simulink model "dc_motor_control_PCI_16E4_2015a"  (R2020b)
settings: Solver=ode3  StartTime=0.0  StopTime=10  RelTol=1e-3
model workspace (MAT data in the model file):
  freq = 0
  tau = 1.51
values from neighbouring files (symbols this model uses):
  a = 37.04    [ControlSystemDesigner_e_Nyquist.m]    (also in ex3_5.m)
  k0 = 1.382    [ControlSystemDesigner_e_Nyquist.m]
  k1 = 6.9094    [ControlSystemDesigner_e_Nyquist.m]
  z = 14.89    [ControlSystemDesigner_e_Nyquist.m]    (also in ex3_5.m = 5)
undefined symbols (not defined in the file or in its folder): National_Instruments, PCI
libraries: sldrtlib x5
settings Model: SimulationMode=external  ExtModeTrigDuration=60001  Creator=Alunos  LastModifiedBy=rodsc
settings DataIOCC: LimitDataPoints=on  SaveFormat=Array  ReturnWorkspaceOutputs=off
settings OptimizationCC: BlockReduction=off  BooleanDataType=off
settings DebuggingCC: SaveWithParameterizedLinksMsg=none  UnderspecifiedInitializationDetection=Classic  MergeDetectMultiDrivingBlocksExec=none  SignalResolutionControl=TryResolveAllWithWarning  SFUnexpectedBacktrackingDiag=warning  SFNoUnconditionalDefaultTransitionDiag=warning  SFExecutionAtInitializationDiag=none  ArithmeticOperatorsInVariantConditions=warning
settings HardwareCC: TargetIntDivRoundTo=Zero  TargetEndianess=LittleEndian  TargetHWDeviceType=Intel->x86/Pentium
settings ModelReferenceCC: PropagateSignalLabelsOutOfModel=off
settings SFSimCC: SimUseLocalCustomCode=off  CustomCodeUndefinedFunction=UseInterfaceOnly
settings RTWCC: Description=Simulink Desktop Real-Time  SystemTargetFile=sldrt.tlc  TemplateMakefile=sldrt.tmf  RTWUseLocalCustomCode=off  RTWCompilerOptimization=on
settings CodeAppCC: MaxIdLength=95  StateflowObjectComments=on
settings SimulinkDesktopRealTimeCC: TargetPreCompLibLocation=C:\Program Files\Matlab\toolbox\sldrt\lib\win64  TargetLangStandard=C89/C90 (ANSI)  SupportVariableSizeSignals=off
settings ConfigComp: CovMetricSettings=dw  CovSaveCumulativeToWorkspaceVar=on  CovSaveSingleToWorkspaceVar=on  CovExternalEMLEnable=off

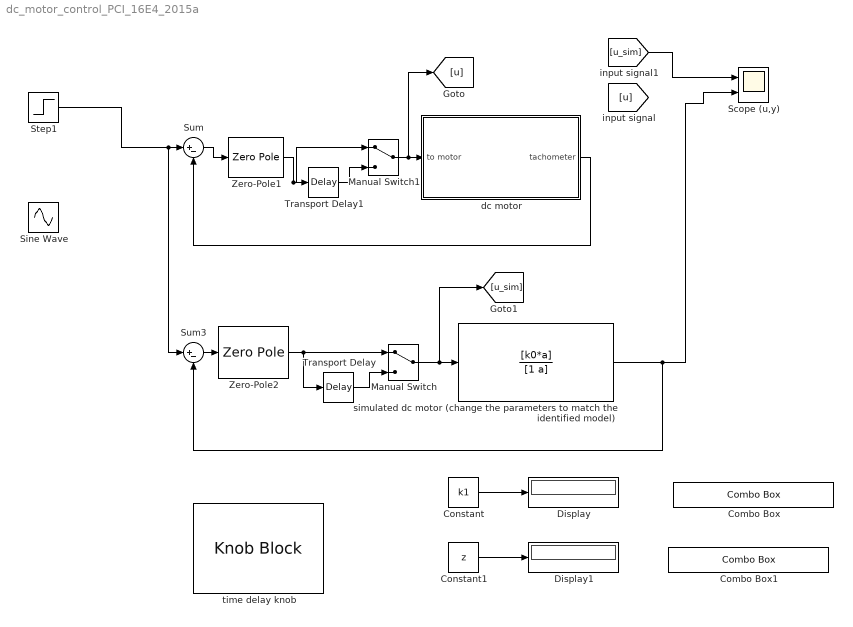
== system dc_motor_control_PCI_16E4_2015a ==
  Combo Box : ComboBox  LabelPosition=Hide  SelectedLabel=Label3
      settings: Values={{'Label1', 'Label2', 'Label3', 'default'}, [4 30 800 6.9094]}
  Combo Box1 : ComboBox  LabelPosition=Hide  SelectedLabel=Label2
      settings: Values={{'Label1', 'Label2', 'Label3', 'default'}, [4 50 150 14.89]}
  Constant : Constant  Value=k1
  Constant1 : Constant  Value=z
  Display : Display
  Display1 : Display
  Manual Switch : ManualSwitch
  Manual Switch1 : ManualSwitch
  Scope (u,y) : Scope  NumInputPorts=2
  Sine Wave : Sin  SampleTime=0
  Step1 : Step  Time=0.2  SampleTime=0
  Sum : Sum  Inputs=|+-
  Sum3 : Sum  Inputs=|+-
  Transport Delay : TransportDelay  DelayTime=tau  FixedBuffer=on  TransDelayFeedthrough=on
  Transport Delay1 : TransportDelay  DelayTime=tau  FixedBuffer=on  TransDelayFeedthrough=on
  Zero-Pole1 : ZeroPole  Zeros=[-z]  Poles=[0]  Gain=[k1/z]
  Zero-Pole2 : ZeroPole  Zeros=[-z]  Poles=0  Gain=[k1/z]
  dc motor : Subsystem
  simulated dc motor (change the parameters to match the identified model) : TransferFcn  Numerator=[k0*a]  Denominator=[1 a]
  time delay knob : KnobBlock  ScaleMax=0.150  TickInterval=0.1
  wires:
  simulated dc motor (change the parameters to match the identified model)/1 -> Scope (u,y)/2, Sum3/2
  Sum/1 -> Zero-Pole1/1
  Zero-Pole2/1 -> Transport Delay/1, Manual Switch/1
  [u_sim] -> Scope (u,y)/1
  Sum3/1 -> Zero-Pole2/1
  dc motor/1(tachometer) -> Sum/2
  Manual Switch/1 -> [u_sim], simulated dc motor (change the parameters to match the identified model)/1
  Transport Delay/1 -> Manual Switch/2
  Zero-Pole1/1 -> Manual Switch1/1, Transport Delay1/1
  Transport Delay1/1 -> Manual Switch1/2
  Manual Switch1/1 -> [u], dc motor/1(to motor)
  Step1/1 -> Sum3/1, Sum/1
  Constant1/1 -> Display1/1
  Constant/1 -> Display/1

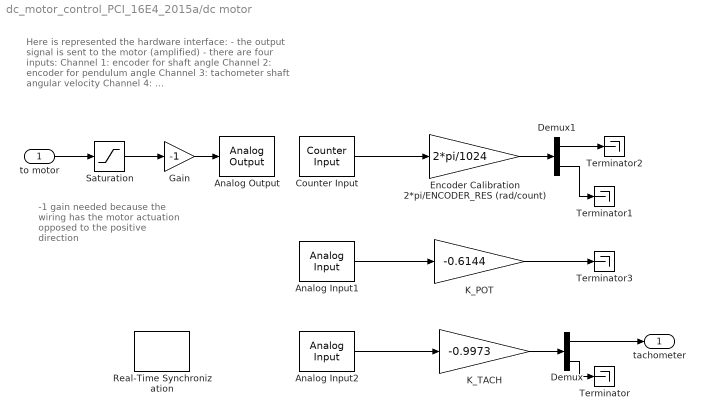
== system dc_motor_control_PCI_16E4_2015a/dc motor ==
  note: -1 gain needed
      | because the wiring
      | has the motor
      | actuation opposed to
      | the positive direction
  note: Here is represented the hardware interface:
      | - the output signal is sent to the motor (amplified)
      | - there are four inputs:
      | Channel 1: encoder for shaft angle
      | Channel 2: encoder for pendulum angle
      | Channel 3: tachometer shaft angular velocity
      | Channel 4: ...
  to motor : Inport
  Analog Input1 : sldrtlib/Analog Input  SampleTime=0.001  MaxMissedTicks=10  ShowMissedTicks=off  YieldWhenWaiting=off  DrvName=National_Instruments/PCI-6221  DrvAddress=4294967295  DrvOptions=[0 0 0 0 0]  Channels=1:2  RangeMode=1  VoltRange=1  DataType=1
      settings: AttributesFormatString=National Instruments\nPCI-6221 [auto]
  Analog Input2 : sldrtlib/Analog Input  SampleTime=0.001  MaxMissedTicks=10  ShowMissedTicks=off  YieldWhenWaiting=off  DrvName=National_Instruments/PCI-6221  DrvAddress=4294967295  DrvOptions=[0 0 0 0 0]  Channels=3:4  RangeMode=1  VoltRange=1  DataType=1
      settings: AttributesFormatString=National Instruments\nPCI-6221 [auto]
  Analog Output : sldrtlib/Analog Output  SampleTime=0.001  MaxMissedTicks=inf  ShowMissedTicks=off  YieldWhenWaiting=off  DrvName=National_Instruments/PCI-6221  DrvAddress=4294967295  DrvOptions=[0 0 0 0 0]  Channels=1  RangeMode=1  VoltRange=1  InitialValue=[]  FinalValue=0
      settings: AttributesFormatString=National Instruments\nPCI-6221 [auto]
  Counter Input : sldrtlib/Counter Input  SampleTime=0.001  MaxMissedTicks=inf  ShowMissedTicks=off  YieldWhenWaiting=off  DrvName=National_Instruments/PCI-6221  DrvAddress=4294967295  DrvOptions=[0 0 0 0 0]  Channels=1:2  ResetMode=1  CounterEdge=1  CounterGate=1  DataType=1
      settings: AttributesFormatString=National Instruments\nPCI-6221 [auto]  SourceProductBaseCode=WT
  Demux : Demux  Outputs=2
  Demux1 : Demux  Outputs=2
  Encoder Calibration 2*pi/ENCODER_RES (rad/count) : Gain  Gain=2*pi/1024  SaturateOnIntegerOverflow=on  OutDataTypeStr=Inherit: Same as input  ParamDataTypeStr=Inherit: Same as input
  Gain : Gain  Gain=-1
  K_POT : Gain  Gain=-0.6144  SaturateOnIntegerOverflow=on  OutDataTypeStr=Inherit: Same as input  ParamDataTypeStr=Inherit: Same as input
  "K_TACH " : Gain  Gain=-0.9973  SaturateOnIntegerOverflow=on  OutDataTypeStr=Inherit: Same as input  ParamDataTypeStr=Inherit: Same as input
  Real-Time Synchronization : sldrtlib/Real-Time Synchronization  SampleTime=0.001  MaxMissedTicks=inf  ShowMissedTicks=off  YieldWhenWaiting=off
  Saturation : Saturate  UpperLimit=5  LowerLimit=-5
  Terminator{,1..3} (4 alike) : Terminator
  tachometer : Outport
  wires:
  Analog Input1/1 -> K_POT/1
  Gain/1 -> Analog Output/1
  Counter Input/1 -> Encoder Calibration 2*pi/ENCODER_RES (rad/count)/1
  Analog Input2/1 -> "K_TACH "/1
  K_POT/1 -> Terminator3/1
  "K_TACH "/1 -> Demux/1
  Demux/1 -> tachometer/1
  Demux/2 -> Terminator/1
  to motor/1 -> Saturation/1
  Saturation/1 -> Gain/1
  Demux1/2 -> Terminator1/1
  Encoder Calibration 2*pi/ENCODER_RES (rad/count)/1 -> Demux1/1
  Demux1/1 -> Terminator2/1
